simulink model "initial_model1"  (R2017b)
settings: Solver=ode4  StartTime=0.0  StopTime=time_final  FixedStep=time_step  RelTol=1e-3  AbsTol=1e-6
values from neighbouring files (symbols this model uses):
  A_frontal = 2.8    [tesla_sim_data1.m]
  C_d = 0.24    [tesla_sim_data1.m]
  enable_stop = 1    [tesla_sim_data1.m]
  ess_cap_scale = 1    [tesla_sim_data1.m]
  ess_fixtemp = 25    [tesla_sim_data1.m]
  ess_init_soc = soc_init_index(simrun)    [ev_sim_init1.m]
  ess_max_ah_cap = ess_max_kwhr_cap*1000/350*[1 1]    [tesla_sim_data1.m]
  ess_max_volts = 9    [tesla_sim_data1.m]
  ess_min_volts = 6    [tesla_sim_data1.m]
  ess_module_num = 40    [tesla_sim_data1.m]
  ess_r_chg = [ ... (first row only)    [tesla_sim_data1.m]
  ess_r_dis = [ ... (first row only)    [tesla_sim_data1.m]
  ess_res_scale_coef = [1 0 1 0]    [tesla_sim_data1.m]
  ess_res_scale_fun = inline('(x(1)*ess_module_num+x(2))/(x(3)*ess_cap_scale+x(4))','x','ess_module_num','ess_cap_scale')    [tesla_sim_data1.m]
  ess_soc = [0 0.1 0.2 0.3 0.4 0.5 0.6 0.7 0.8 0.9 1]    [tesla_sim_data1.m]
  ess_tmp = [0 25]    [tesla_sim_data1.m]
  ess_voc = [ ... (first row only)    [tesla_sim_data1.m]
  f_rolling = 0.018    [tesla_sim_data1.m]
  FR = 9.73    [tesla_sim_data1.m]
  g_gravity = 9.81    [tesla_sim_data1.m]
  K_factor_in = 2    [ev_sim_init1.m]
  Kp_c = 30    [ev_sim_init1.m]
  m_map_spd = [0	100	250	500	1000	1500	2000	2500	3000	4000	4500	5500	6000	7000	8000	9000	10000]*(2*pi)/60    [tesla_sim_data1.m]
  m_max_trq_IM = min(m_peak_trq_IM, m_peak_pwr*1000./m_map_spd)    [tesla_sim_data1.m]
  m_max_trq_SR = min(m_peak_trq_SR, m_peak_pwr*1000./m_map_spd)    [tesla_sim_data1.m]
  m_min_volts = 200    [tesla_sim_data1.m]
  m_peak_pwr = 310    [tesla_sim_data1.m]
  M_total = (4650+300)/2.2046    (= 2245.3052708)    [tesla_sim_data1.m]
  p00 = -215.8    [tesla_sim_data1.m]
  p01 = 3.368    [tesla_sim_data1.m]
  p02 = -0.0178    [tesla_sim_data1.m]
  p03 = 6.515e-05    [tesla_sim_data1.m]
  p10 = 4.164    [tesla_sim_data1.m]
  p11 = 0.04408    [tesla_sim_data1.m]
  p12 = 9.874e-05    [tesla_sim_data1.m]
  p20 = -0.009417    [tesla_sim_data1.m]
  p21 = 5.981e-06    [tesla_sim_data1.m]
  p30 = 5.161e-06    [tesla_sim_data1.m]
  R_tire = 0.335    [tesla_sim_data1.m]
  regstop_soc = 0.9    [ev_sim_init1.m]
  rho_air = 1.2    [tesla_sim_data1.m]
  Ti_c = 60    [ev_sim_init1.m]
  time_final = 1*length(cyc_mph(:,2))    [ev_sim_init1.m]
  Tt_c = 65    [ev_sim_init1.m]
  v_max_c = 100    [ev_sim_init1.m]
undefined symbols (not defined in the file or in its folder): cyc_mph
libraries: simulink x4
settings Model: ExtModeTrigMode=oneshot  ExtModeArmWhenConnect=off  Creator=sz3lhr  LastModifiedBy=Robert Wygant
settings SolverCC: InitialStep=0.001
settings DataIOCC: SaveFormat=Array  SignalLoggingSaveFormat=ModelDataLogs  SaveOutput=off  SaveTime=off  SignalLoggingName=sigsOut
settings OptimizationCC: BooleanDataType=off  OptimizeBlockIOStorage=off  BufferReuse=off  GlobalBufferReuse=off  ExpressionFolding=off  ExpressionDepthLimit=2147483647  LocalBlockOutputs=off  InitFltsAndDblsToZero=on  LifeSpan=inf
settings DebuggingCC: SaveWithParameterizedLinksMsg=none  UnderspecifiedInitializationDetection=Classic  MergeDetectMultiDrivingBlocksExec=none  SignalResolutionControl=TryResolveAllWithWarning  MultiTaskDSMMsg=warning  MultiTaskCondExecSysMsg=none  FcnCallInpInsideContextMsg=warning  StateNameClashWarn=warning  StrictBusMsg=None  SFUnexpectedBacktrackingDiag=warning  SFNoUnconditionalDefaultTransitionDiag=warning  SFExecutionAtInitializationDiag=none
settings HardwareCC: ProdBitPerPointer=32  ProdBitPerSizeT=32  ProdBitPerPtrDiffT=32  ProdLargestAtomicFloat=None  ProdIntDivRoundTo=Undefined  ProdEndianess=Unspecified  ProdWordSize=32  ProdHWDeviceType=32-bit Generic  TargetUnknown=on
settings ModelReferenceCC: PropagateSignalLabelsOutOfModel=off
settings CodeAppCC: StateflowObjectComments=on
settings GRTTargetCC: TargetFcnLib=ansi_tfl_tmw.mat  TargetLangStandard=C89/C90 (ANSI)  GeneratePreprocessorConditionals=Disable all  CombineOutputUpdateFcns=off  GRTInterface=on
settings ConfigComp: CovMetricSettings=dw  CovHtmlReporting=on  CovSaveCumulativeToWorkspaceVar=on  CovSaveSingleToWorkspaceVar=on  CovExternalEMLEnable=off

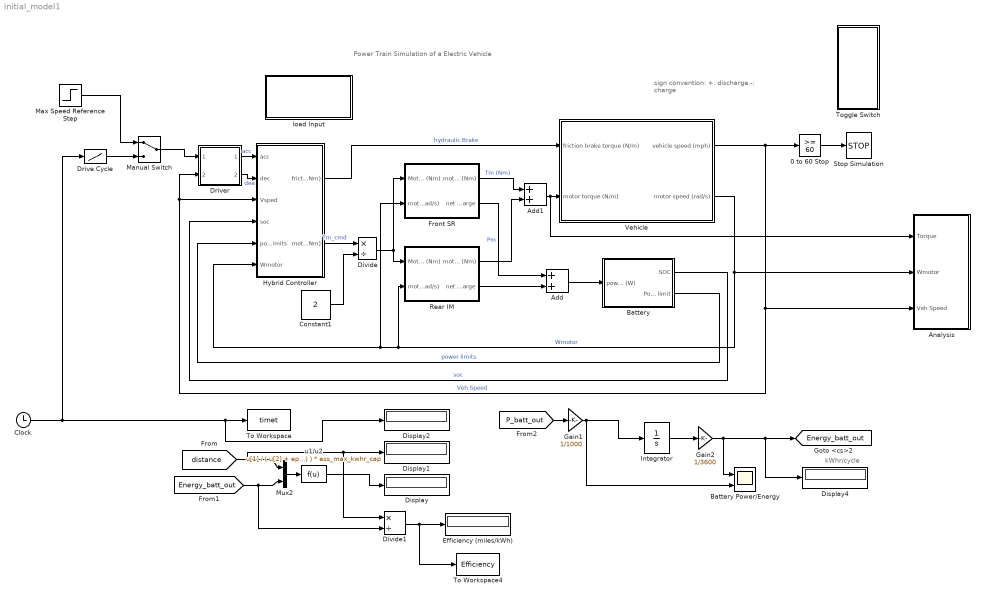
== system initial_model1 ==
  note: Power Train Simulation of a Electric Vehicle
  note: sign convention:
      | +: discharge     -: charge
  note: kWhr/cycle
  0 to 60 Stop : simulink/Logic and Bit Operations/Compare To Constant  relop=>=  const=60  OutDataTypeStr=boolean
  Add : Sum
  Add1 : Sum
  Analysis : Subsystem
  Battery : Subsystem
      mask Display: disp('Battery')
  Battery Power/Energy : Scope  NumInputPorts=2
      settings: Description=Power/Energy
  Clock : Clock
  Constant1 : Constant  Value=2  VectorParams1D=off  SampleTime=-1
  Display{,1..2,4} (4 alike) : Display
  Divide : Product  Inputs=*/
  Divide1 : Product  Inputs=*/
  Drive Cycle : Lookup  InputValues=cyc_mph(:,1)  Table=cyc_mph(:,2)  SaturateOnIntegerOverflow=on
  "Driver " : Subsystem
      mask Display: disp('Driver')
  Efficiency (miles/kWh) : Display
  Front SR : Subsystem
      mask Display: disp('Electric\nMotor')
  Gain1 : Gain  Gain=1/1000  SaturateOnIntegerOverflow=on  OutDataTypeStr=Inherit: Same as input  ParamDataTypeStr=Inherit: Same as input
  Gain2 : Gain  Gain=1/3600  SaturateOnIntegerOverflow=on  OutDataTypeStr=Inherit: Same as input  ParamDataTypeStr=Inherit: Same as input
  Hybrid Controller : Subsystem
      mask Display: disp('Vehicle\nController')
  Integrator : Integrator  LowerSaturationLimit=0
  Manual Switch : ManualSwitch
  Max Speed Reference Step : Step  Time=0.01  After=500  SampleTime=0
  Mux2 : Mux  Inputs=2
  Rear IM : Subsystem
      mask Display: disp('Electric\nMotor')
  Stop Simulation : Stop
  To Workspace : ToWorkspace  VariableName=timet  SampleTime=-1
  To Workspace4 : ToWorkspace  VariableName=Efficiency  SampleTime=-1
      settings: Save2DSignal=2-D array (concatenate along first dimension)
  Toggle Switch : Subsystem  DialogController=hmiCreateDDGDialog  IsWebBlock=on  mask(MWDashboardBlock){webBlockId=bcc0d4d4-d3e6-44b1-9da5-97979c717e77, webBlockType=toggleswitch, ShowInLibBrowser=on, ShowInitialText=on, HMISrcModelName=initial_model1}
      mask prompts: webBlockId "WebBlock Id"; webBlockType "WebBlock Type"; HMISrcModelName "Source Model"
      mask help: SimulinkHMI:dialogs:SwitchDialogDesc
      mask Help: helpview([docroot '/mapfiles/simulink.map'], 'hmi_toggle_switch')
      mask Display:
      | if strcmp(get_param(bdroot(gcb),'BlockDiagramType'), 'library')
      |     image([(matlabroot) '/toolbox/simulink/hmi/icons/ToggleSwitch.png']);
      | end
  Vehicle : Subsystem
      mask Display: disp('Vehicle \nDynamic Model')
  load Input : Subsystem
      settings: OpenFcn=ev_sim_init
      mask Help: This block runs/ndes_init.m file in the main directory
      mask Display: disp('Load Input Data\nRun Simulation')
  u1/u2 : Fcn  Expr=u[1] / ( u[2] + eps*(u[2] == 0) ) * ess_max_kwhr_cap
  tag scope: Energy_batt_out=global
  wires:
  Battery/1(SOC) -> Hybrid Controller/4(soc)  "soc"
  Hybrid Controller/1(friction brake torque (Nm)) -> Vehicle/1(friction brake torque (N/m))  "hydraulic Brake"
  Vehicle/1(vehicle speed (mph)) -> 0 to 60 Stop/1, Analysis/3(Veh Speed), Hybrid Controller/3(Vsped), "Driver "/2(Velocity (mph))  "Veh Speed"
  "Driver "/1(Accel Comd) -> Hybrid Controller/1(acc)  "acc"
  "Driver "/2(Brake Comd) -> Hybrid Controller/2(dec)  "dea"
  Vehicle/2(motor speed (rad/s)) -> Analysis/2(Wmotor), Rear IM/2(motor speed (rad/s)), Front SR/2(motor speed (rad/s)), Hybrid Controller/6(Wmotor)  "Wmotor"
  Battery/2(Power limit) -> Hybrid Controller/5(power limits)  "power limits"
  Clock/1 -> Drive Cycle/1, To Workspace/1, Display2/1
  [distance] -> Divide1/1, Display1/1, Mux2/1
  [Energy_batt_out] -> Divide1/2, Mux2/2
  u1/u2/1 -> Display/1
  Mux2/1 -> u1/u2/1
  [P_batt_out] -> Gain1/1
  Gain1/1 -> Integrator/1, Battery Power/Energy/2
  Integrator/1 -> Gain2/1
  Gain2/1 -> [Energy_batt_out], Display4/1, Battery Power/Energy/1
  0 to 60 Stop/1 -> Stop Simulation/1
  Add/1 -> Battery/1(power req'd into bus (W))
  Rear IM/2(net Power >0 discharge <0 charge) -> Add/2
  Front SR/2(net Power >0 discharge <0 charge) -> Add/1  "Pm"
  Rear IM/1(motor torque output (Nm)) -> Add1/2
  Front SR/1(motor torque output (Nm)) -> Add1/1  "Tm (Nm)"
  Hybrid Controller/2(motor torque command (Nm)) -> Divide/1  "Tm_cmd"
  Constant1/1 -> Divide/2
  Divide/1 -> Rear IM/1(Motor demand Torque (Nm)), Front SR/1(Motor demand Torque (Nm))
  Add1/1 -> Analysis/1(Torque), Vehicle/2(motor torque (N/m))
  Max Speed Reference Step/1 -> Manual Switch/1
  Drive Cycle/1 -> Manual Switch/2
  Manual Switch/1 -> "Driver "/1(speed_desired)
  Divide1/1 -> To Workspace4/1, Efficiency (miles/kWh)/1

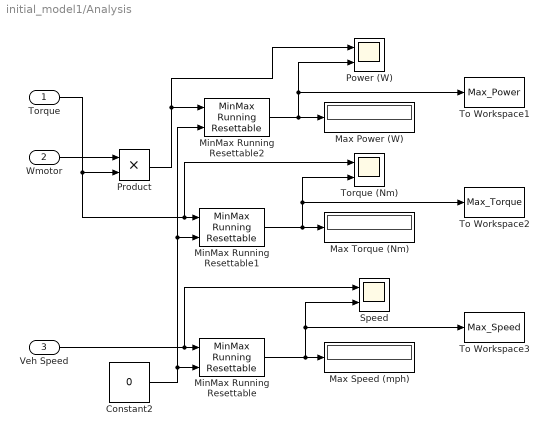
== system initial_model1/Analysis ==
  Torque : Inport
  Wmotor : Inport  Port=2
  Veh Speed : Inport  Port=3
  Constant2 : Constant  Value=0  VectorParams1D=off  SampleTime=-1
  Max Power (W) : Display
  Max Speed (mph) : Display
  Max Torque (Nm) : Display
  MinMax Running Resettable : simulink/Math Operations/MinMax Running Resettable  Function=max  vinit=0.0
  MinMax Running Resettable1 : simulink/Math Operations/MinMax Running Resettable  Function=max  vinit=0.0
  MinMax Running Resettable2 : simulink/Math Operations/MinMax Running Resettable  Function=max  vinit=0.0
  Power (W) : Scope  NumInputPorts=2
  Product : Product
  Speed : Scope  NumInputPorts=2
  To Workspace1 : ToWorkspace  VariableName=Max_Power  SampleTime=-1
      settings: Save2DSignal=2-D array (concatenate along first dimension)
  To Workspace2 : ToWorkspace  VariableName=Max_Torque  SampleTime=-1
      settings: Save2DSignal=2-D array (concatenate along first dimension)
  To Workspace3 : ToWorkspace  VariableName=Max_Speed  SampleTime=-1
      settings: Save2DSignal=2-D array (concatenate along first dimension)
  Torque (Nm) : Scope  NumInputPorts=2
  wires:
  Veh Speed/1 -> Speed/1, MinMax Running Resettable/1
  Wmotor/1 -> Product/1
  Torque/1 -> Torque (Nm)/1, MinMax Running Resettable1/1, Product/2
  Product/1 -> MinMax Running Resettable2/1, Power (W)/1
  Constant2/1 -> MinMax Running Resettable2/2, MinMax Running Resettable1/2, MinMax Running Resettable/2
  MinMax Running Resettable1/1 -> To Workspace2/1, Torque (Nm)/2, Max Torque (Nm)/1
  MinMax Running Resettable/1 -> To Workspace3/1, Speed/2, Max Speed (mph)/1
  MinMax Running Resettable2/1 -> To Workspace1/1, Power (W)/2, Max Power (W)/1

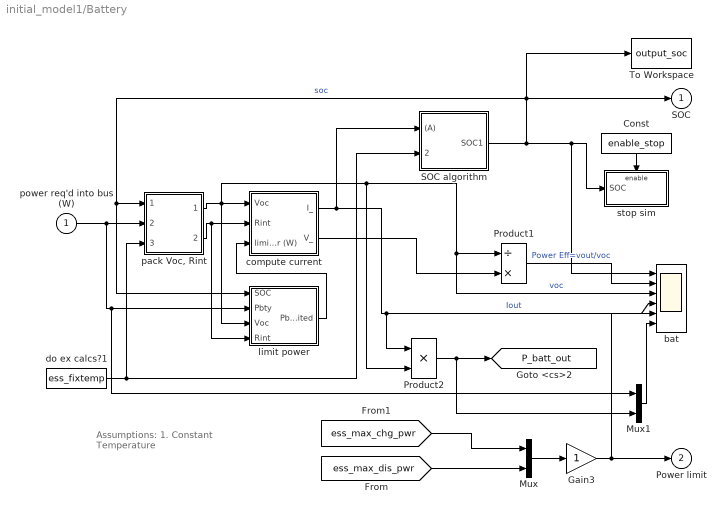
== system initial_model1/Battery ==
  note: Assumptions:
      | 1. Constant Temperature
  power req'd into bus (W) : Inport
  Const : Constant  Value=enable_stop
  Gain3 : Gain  SaturateOnIntegerOverflow=on  OutDataTypeStr=Inherit: Same as input  ParamDataTypeStr=Inherit: Same as input
  Mux : Mux  Inputs=2
  Mux1 : Mux  Inputs=2
  Product1 : Product  Inputs=/*  SaturateOnIntegerOverflow=on  InputSameDT=on  OutDataTypeStr=Inherit: Same as first input
  Product2 : Product  Inputs=**  SaturateOnIntegerOverflow=on  InputSameDT=on  OutDataTypeStr=Inherit: Same as first input
  SOC algorithm : Subsystem  AncestorBlock=|
      | lib_energy_storage/Ess Choices/energy
      | storage <ess>/SOC
      | algorithm
      mask Display: disp('SOC\nalgorithm')
  To Workspace : ToWorkspace  VariableName=output_soc  SampleTime=-1
  bat : Scope  NumInputPorts=6
  compute current : Subsystem  AncestorBlock=|
      | lib_energy_storage/Ess Choices/energy
      | storage <ess>/compute
      | current
      mask Display: disp('Compute\nCurrent')
  do ex calcs?1 : Constant  Value=ess_fixtemp
  limit power : Subsystem  AncestorBlock=lib_energy_storage/Ess Choices/energy storage <ess>/limit power
      mask Display: disp('Limit\nPower')
  "pack Voc, Rint" : Subsystem  AncestorBlock=|
      | lib_energy_storage/Ess Choices/energy
      | storage <ess>/pack
      | Voc, Rint
      mask Display: disp('Pack\nVoc,Rint')
  stop sim : Subsystem  AncestorBlock=lib_energy_storage/Ess Choices/energy storage <ess>/stop sim  TreatAsAtomicUnit=on
  SOC : Outport  InitialOutput=0
  Power limit : Outport  Port=2  InitialOutput=0
  tag scope: P_batt_out=global
  wires:
  limit power/1("Pbty, limited") -> compute current/3(limited output power (W))
  "pack Voc, Rint"/1(pack open- circuit voltage) -> limit power/3(Voc), compute current/1(Voc), Product1/1, bat/3, Product2/2  "voc"
  "pack Voc, Rint"/2(pack resistance) -> compute current/2(Rint), limit power/4(Rint)
  Const/1 -> stop sim/Enable
  SOC algorithm/1(SOC1) -> limit power/1(SOC), "pack Voc, Rint"/1(SOC (prev)), SOC/1, To Workspace/1, stop sim/1(SOC), bat/1  "soc"
  compute current/1(I_) -> SOC algorithm/1((A)), Product2/1, bat/4  "Iout"
  power req'd into bus (W)/1 -> "pack Voc, Rint"/2(req'd battery power (W)), limit power/2(Pbty), Mux1/1
  compute current/2(V_) -> Product1/2
  do ex calcs?1/1 -> "pack Voc, Rint"/3(mod tmp (C)), SOC algorithm/2(tmp (C))
  Mux/1 -> Gain3/1
  Product1/1 -> bat/2  "Power Eff=vout/voc"
  [ess_max_dis_pwr] -> Mux/2
  [ess_max_chg_pwr] -> Mux/1
  Gain3/1 -> Power limit/1, bat/5
  Product2/1 -> [P_batt_out], Mux1/2
  Mux1/1 -> bat/6

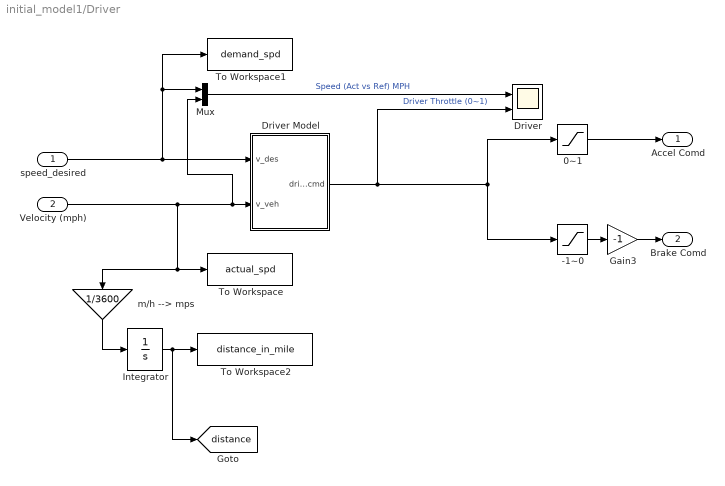
== system initial_model1/Driver  ==
  speed_desired : Inport
  Velocity (mph) : Inport  Port=2
  -1~0 : Saturate  UpperLimit=0  LowerLimit=-1
  0~1 : Saturate  UpperLimit=1  LowerLimit=0
  Driver : Scope  NumInputPorts=2
  Driver Model : Subsystem
  Gain3 : Gain  Gain=-1  SaturateOnIntegerOverflow=on  OutDataTypeStr=Inherit: Same as input  ParamDataTypeStr=Inherit: Same as input
  Integrator : Integrator  LowerSaturationLimit=0
  Mux : Mux  Inputs=2
  To Workspace : ToWorkspace  VariableName=actual_spd  SampleTime=-1
  To Workspace1 : ToWorkspace  VariableName=demand_spd  SampleTime=-1
  To Workspace2 : ToWorkspace  VariableName=distance_in_mile  SampleTime=time_final
  m/h --> mps : Gain  Gain=1/3600  SaturateOnIntegerOverflow=on  OutDataTypeStr=Inherit: Same as input  ParamDataTypeStr=Inherit: Same as input
  Accel Comd : Outport  InitialOutput=0
  Brake Comd : Outport  Port=2  InitialOutput=0
  tag scope: distance=global
  wires:
  speed_desired/1 -> Driver Model/1(v_des), To Workspace1/1, Mux/1
  Velocity (mph)/1 -> To Workspace/1, m/h --> mps/1, Driver Model/2(v_veh), Mux/2
  Driver Model/1(driver_cmd) -> Driver/2, 0~1/1, -1~0/1  "Driver Throttle (0~1)"
  -1~0/1 -> Gain3/1
  0~1/1 -> Accel Comd/1
  Gain3/1 -> Brake Comd/1
  Mux/1 -> Driver/1  "Speed (Act vs Ref) MPH"
  Integrator/1 -> To Workspace2/1, [distance]
  m/h --> mps/1 -> Integrator/1

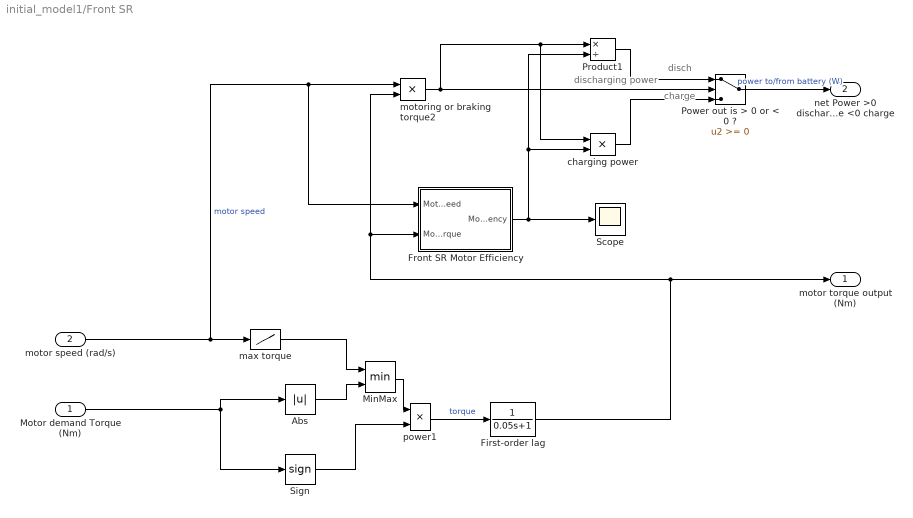
== system initial_model1/Front SR ==
  note: disch
  note: charge
  note: discharging
      | power
  Motor demand Torque (Nm) : Inport
  motor speed (rad/s) : Inport  Port=2
  Abs : Abs  SaturateOnIntegerOverflow=on
  First-order lag : TransferFcn  Denominator=[0.05 1]
  Front SR Motor Efficiency : Subsystem
      mask Display:
      | color('green')
      | disp("Motor Efficiency")
  MinMax : MinMax  Inputs=2  SaturateOnIntegerOverflow=on  InputSameDT=on
  Power out is > 0 or < 0 ? : Switch  SaturateOnIntegerOverflow=on  InputSameDT=on
  Product1 : Product  Inputs=*/  SaturateOnIntegerOverflow=on  InputSameDT=on  OutDataTypeStr=Inherit: Same as first input
  Scope : Scope
  Sign : Signum
  charging power : Product  SaturateOnIntegerOverflow=on  InputSameDT=on  OutDataTypeStr=Inherit: Same as first input
  max torque : Lookup  InputValues=m_map_spd  Table=m_max_trq_SR  SaturateOnIntegerOverflow=on
  motoring or braking torque2 : Product  SaturateOnIntegerOverflow=on  InputSameDT=on  OutDataTypeStr=Inherit: Same as first input
  power1 : Product  SaturateOnIntegerOverflow=on  InputSameDT=on  OutDataTypeStr=Inherit: Same as first input
  motor torque output (Nm) : Outport  InitialOutput=0
  net Power >0 discharge <0 charge : Outport  Port=2  InitialOutput=0
  wires:
  charging power/1 -> Power out is > 0 or < 0 ?/3
  Product1/1 -> Power out is > 0 or < 0 ?/1
  Power out is > 0 or < 0 ?/1 -> net Power >0 discharge <0 charge/1  "power to/from battery (W)"
  Motor demand Torque (Nm)/1 -> Sign/1, Abs/1
  power1/1 -> First-order lag/1  "torque"
  motoring or braking torque2/1 -> Product1/1, charging power/1, Power out is > 0 or < 0 ?/2
  Abs/1 -> MinMax/2
  MinMax/1 -> power1/1
  Sign/1 -> power1/2
  motor speed (rad/s)/1 -> max torque/1, Front SR Motor Efficiency/1(Motor_speed), motoring or braking torque2/1  "motor speed"
  First-order lag/1 -> motor torque output (Nm)/1, Front SR Motor Efficiency/2(Motor_torque), motoring or braking torque2/2
  max torque/1 -> MinMax/1
  Front SR Motor Efficiency/1(Motor_efficiency) -> Scope/1, charging power/2, Product1/2

== system initial_model1/Hybrid Controller ==
  acc : Inport
  dec : Inport  Port=2
  Vsped : Inport  Port=3
  soc : Inport  Port=4
  power limits : Inport  Port=5
  Wmotor : Inport  Port=6
  Brake : Subsystem  AncestorBlock=|
      | lib_controls/<vc> prius/Coordinated
      |  Controller/max engine
      | efficiency point
      mask Display: disp('Braking\nControl')
  Demux : Demux  Outputs=2
  Drive : Subsystem  AncestorBlock=|
      | lib_controls/<vc> prius/Coordinated
      |  Controller/max engine
      | efficiency point
      mask Display: disp('Driving\nControl')
  Mux : Mux  Inputs=2
  Mux1 : Mux  Inputs=2
  power >=0 drive <0 brake : Switch  SaturateOnIntegerOverflow=on
  pwr_demand : Subsystem
      mask Display: disp('Power\nDemand')
  friction brake torque (Nm) : Outport
  motor torque command (Nm) : Outport  Port=2
  wires:
  pwr_demand/1(pwr dmd (W)) -> Drive/1(pwr requested), Brake/1(Driver power requested (W)), power >=0 drive <0 brake/2
  acc/1 -> pwr_demand/1(Accel cmd)
  dec/1 -> pwr_demand/2(Decel cmd)
  Mux/1 -> power >=0 drive <0 brake/1
  Mux1/1 -> power >=0 drive <0 brake/3
  power >=0 drive <0 brake/1 -> Demux/1
  Vsped/1 -> Brake/2(Veh speed (mph))
  soc/1 -> Brake/3(soc)
  power limits/1 -> Brake/4(Power limit (W)), Drive/2(Power limits (W))
  Wmotor/1 -> Brake/5(motor speed(rad/s)), Drive/3(motor speed (rad/s))
  Drive/2(motor torque command (Nm)) -> Mux/2
  Drive/1(friction brake torque (Nm)) -> Mux/1
  Brake/1(friction brake torque command (Nm)) -> Mux1/1
  Brake/2(motor torque command (Nm)) -> Mux1/2
  Demux/2 -> motor torque command (Nm)/1
  Demux/1 -> friction brake torque (Nm)/1

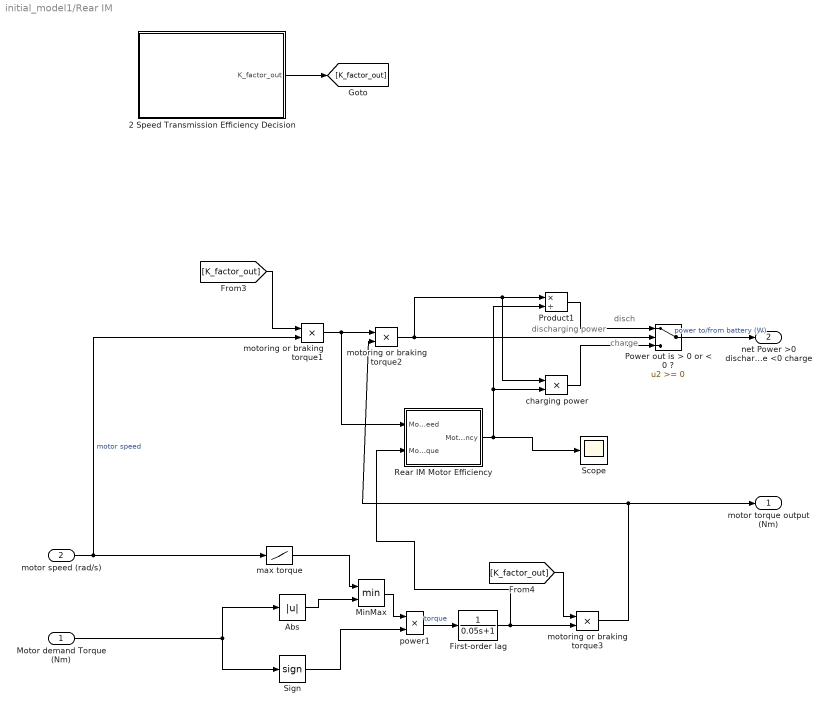
== system initial_model1/Rear IM ==
  note: disch
  note: charge
  note: discharging
      | power
  Motor demand Torque (Nm) : Inport
  motor speed (rad/s) : Inport  Port=2
  2 Speed Transmission Efficiency Decision : Subsystem
  Abs : Abs  SaturateOnIntegerOverflow=on
  First-order lag : TransferFcn  Denominator=[0.05 1]
  MinMax : MinMax  Inputs=2  SaturateOnIntegerOverflow=on  InputSameDT=on
  Power out is > 0 or < 0 ? : Switch  SaturateOnIntegerOverflow=on  InputSameDT=on
  Product1 : Product  Inputs=*/  SaturateOnIntegerOverflow=on  InputSameDT=on  OutDataTypeStr=Inherit: Same as first input
  Rear IM Motor Efficiency : Subsystem
      mask Display:
      | color('green')
      | disp("Motor Efficiency")
  Scope : Scope
  Sign : Signum
  charging power : Product  SaturateOnIntegerOverflow=on  InputSameDT=on  OutDataTypeStr=Inherit: Same as first input
  max torque : Lookup  InputValues=m_map_spd  Table=m_max_trq_IM  SaturateOnIntegerOverflow=on
  motoring or braking torque1 : Product  SaturateOnIntegerOverflow=on  InputSameDT=on  OutDataTypeStr=Inherit: Same as first input
  motoring or braking torque2 : Product  SaturateOnIntegerOverflow=on  InputSameDT=on  OutDataTypeStr=Inherit: Same as first input
  motoring or braking torque3 : Product  SaturateOnIntegerOverflow=on  InputSameDT=on  OutDataTypeStr=Inherit: Same as first input
  power1 : Product  SaturateOnIntegerOverflow=on  InputSameDT=on  OutDataTypeStr=Inherit: Same as first input
  motor torque output (Nm) : Outport  InitialOutput=0
  net Power >0 discharge <0 charge : Outport  Port=2  InitialOutput=0
  wires:
  charging power/1 -> Power out is > 0 or < 0 ?/3
  Product1/1 -> Power out is > 0 or < 0 ?/1
  Power out is > 0 or < 0 ?/1 -> net Power >0 discharge <0 charge/1  "power to/from battery (W)"
  motor speed (rad/s)/1 -> max torque/1, motoring or braking torque1/2  "motor speed"
  Motor demand Torque (Nm)/1 -> Abs/1, Sign/1
  power1/1 -> First-order lag/1  "torque"
  motoring or braking torque2/1 -> Product1/1, charging power/1, Power out is > 0 or < 0 ?/2
  Abs/1 -> MinMax/2
  MinMax/1 -> power1/1
  Sign/1 -> power1/2
  max torque/1 -> MinMax/1
  First-order lag/1 -> Rear IM Motor Efficiency/2(Motor_torque), motoring or braking torque3/2
  motoring or braking torque1/1 -> Rear IM Motor Efficiency/1(Motor_speed), motoring or braking torque2/1
  motoring or braking torque3/1 -> motoring or braking torque2/2, motor torque output (Nm)/1
  2 Speed Transmission Efficiency Decision/1(K_factor_out) -> [K_factor_out]
  [K_factor_out] -> motoring or braking torque1/1
  [K_factor_out] -> motoring or braking torque3/1
  Rear IM Motor Efficiency/1(Motor_efficiency) -> charging power/2, Product1/2, Scope/1

== system initial_model1/Toggle Switch ==

== system initial_model1/Vehicle ==
  friction brake torque (N/m) : Inport
  motor torque (N/m) : Inport  Port=2
  Dynamics : Subsystem
      mask Display: disp('Vehicle \nDynamic Model')
  rad/s --> mph : Gain  Gain=R_tire/1000*0.621371*3600  SaturateOnIntegerOverflow=on  OutDataTypeStr=Inherit: Same as input  ParamDataTypeStr=Inherit: Same as input
  w_r->w_wh : Fcn  Expr=u/FR
  vehicle speed (mph) : Outport
  motor speed (rad/s) : Outport  Port=2
  wires:
  motor torque (N/m)/1 -> Dynamics/2(Tm: motor torque (N/m))
  friction brake torque (N/m)/1 -> Dynamics/3("Tfb: friction brake torque (N/m) ")
  w_r->w_wh/1 -> Dynamics/1(wheel speed (rad/s)), rad/s --> mph/1
  rad/s --> mph/1 -> vehicle speed (mph)/1
  Dynamics/1(motor speed (rad/s)) -> motor speed (rad/s)/1, w_r->w_wh/1

== system initial_model1/load Input ==
  note: double_click to load

== system initial_model1/Battery/SOC algorithm ==
  note: SOC=(Max Ah capacity-Ah used)/Max Ah capacity
  (A) : Inport
  tmp (C) : Inport  Port=2
  (sec->hrs) : Gain  Gain=1/3600  SaturateOnIntegerOverflow=on  OutDataTypeStr=Inherit: Same as input  ParamDataTypeStr=Inherit: Same as input
  0 <= SOC <= 1 : Saturate  UpperLimit=1  LowerLimit=0
  A-h remaining : Sum  Inputs=-+  SaturateOnIntegerOverflow=on  InputSameDT=on  OutDataTypeStr=Inherit: Same as first input
  Ah used : Integrator  InitialConditionSource=external  InitialCondition=(1-ess_init_soc)*ess_max_ah_cap
  Fcn : Fcn  Expr=1/u
  Fcn1 : Fcn  Expr=(1-ess_init_soc)*u
  SOC : Product  SaturateOnIntegerOverflow=on  InputSameDT=on  OutDataTypeStr=Inherit: Same as first input
  max cap : Lookup  InputValues=ess_tmp  Table=ess_max_ah_cap*ess_cap_scale  SaturateOnIntegerOverflow=on
  SOC1 : Outport  InitialOutput=0
  wires:
  (A)/1 -> (sec->hrs)/1
  (sec->hrs)/1 -> Ah used/1
  Ah used/1 -> A-h remaining/1
  Fcn/1 -> SOC/2
  SOC/1 -> 0 <= SOC <= 1/1
  A-h remaining/1 -> SOC/1
  0 <= SOC <= 1/1 -> SOC1/1
  tmp (C)/1 -> max cap/1
  max cap/1 -> A-h remaining/2, Fcn/1, Fcn1/1
  Fcn1/1 -> Ah used/2

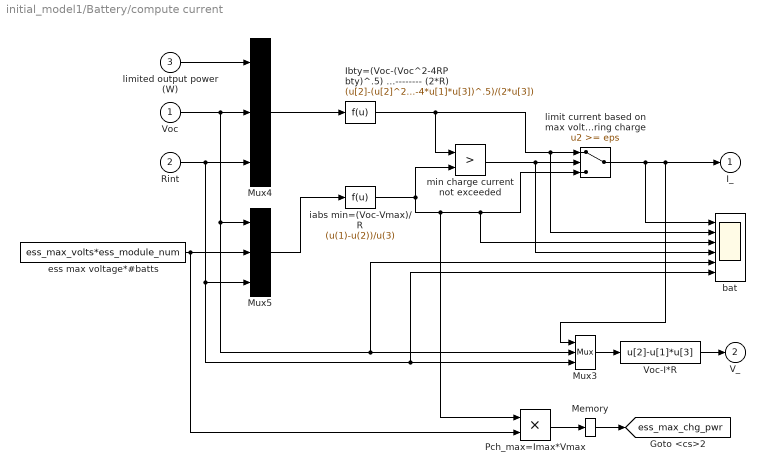
== system initial_model1/Battery/compute current ==
  Voc : Inport
  Rint : Inport  Port=2
  limited output power (W) : Inport  Port=3
  Ibty=(Voc-(Voc^2-4RPbty)^.5) ----------------------------- (2*R) : Fcn  Expr=(u[2]-(u[2]^2-4*u[1]*u[3])^.5)/(2*u[3])
  Memory : Memory
  Mux3 : Mux  Inputs=3
  Mux4 : Mux  Inputs=3
  Mux5 : Mux  Inputs=3
  Pch_max=Imax*Vmax : Product  SaturateOnIntegerOverflow=on  InputSameDT=on  OutDataTypeStr=Inherit: Same as first input
  Voc-I*R : Fcn  Expr=u[2]-u[1]*u[3]
  bat : Scope  NumInputPorts=6
  ess max voltage*#batts : Constant  Value=ess_max_volts*ess_module_num
  iabs min=(Voc-Vmax)/R : Fcn  Expr=(u(1)-u(2))/u(3)
  limit current based on max voltage during charge : Switch  Threshold=eps  SaturateOnIntegerOverflow=on  InputSameDT=on
  min charge current not exceeded : RelationalOperator  Operator=>  RndMeth=Nearest  InputSameDT=on
  I_ : Outport  InitialOutput=0
  V_ : Outport  Port=2  InitialOutput=0
  tag scope: ess_max_chg_pwr=global
  wires:
  limited output power (W)/1 -> Mux4/1
  Voc/1 -> Mux4/2, Mux5/1, Mux3/2, bat/5
  Rint/1 -> Mux4/3, Mux5/3, Mux3/3, bat/6
  Ibty=(Voc-(Voc^2-4RPbty)^.5) ----------------------------- (2*R)/1 -> min charge current not exceeded/1, limit current based on max voltage during charge/1, bat/2
  iabs min=(Voc-Vmax)/R/1 -> min charge current not exceeded/2, Pch_max=Imax*Vmax/1, limit current based on max voltage during charge/3, bat/3
  limit current based on max voltage during charge/1 -> Mux3/1, I_/1, bat/1
  min charge current not exceeded/1 -> limit current based on max voltage during charge/2, bat/4
  Mux3/1 -> Voc-I*R/1
  Voc-I*R/1 -> V_/1
  Mux4/1 -> Ibty=(Voc-(Voc^2-4RPbty)^.5) ----------------------------- (2*R)/1
  Mux5/1 -> iabs min=(Voc-Vmax)/R/1
  ess max voltage*#batts/1 -> Mux5/2, Pch_max=Imax*Vmax/2
  Pch_max=Imax*Vmax/1 -> Memory/1
  Memory/1 -> [ess_max_chg_pwr]

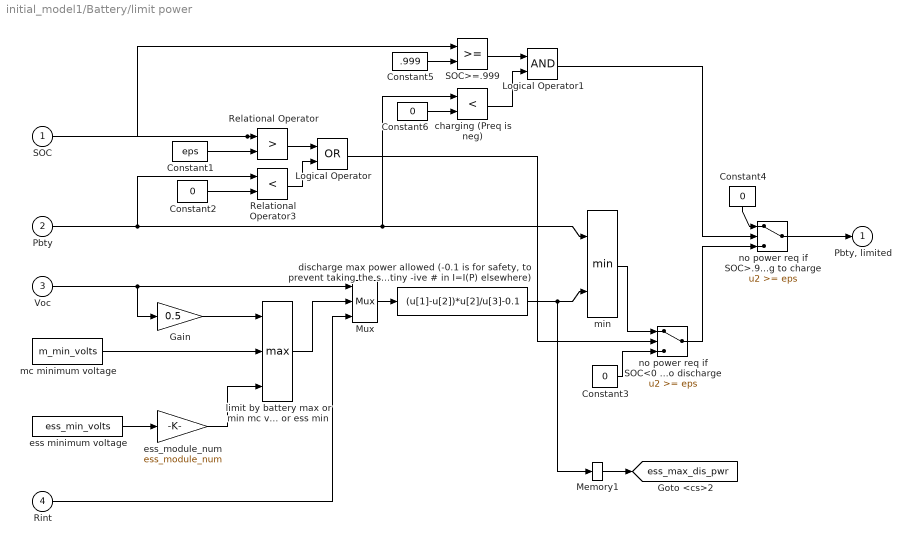
== system initial_model1/Battery/limit power ==
  SOC : Inport
  Pbty : Inport  Port=2
  Voc : Inport  Port=3
  Rint : Inport  Port=4
  Constant1 : Constant  Value=eps
  Constant{2..4,6} (4 alike) : Constant  Value=0
  Constant5 : Constant  Value=.999
  Gain : Gain  Gain=0.5  SaturateOnIntegerOverflow=on  OutDataTypeStr=Inherit: Same as input  ParamDataTypeStr=Inherit: Same as input
  Logical Operator : Logic  Operator=OR
  Logical Operator1 : Logic
  Memory1 : Memory
  Mux : Mux  Inputs=3
  Relational Operator : RelationalOperator  Operator=>  RndMeth=Nearest  InputSameDT=on
  Relational Operator3 : RelationalOperator  Operator=<  RndMeth=Nearest  InputSameDT=on
  SOC>=.999 : RelationalOperator  RndMeth=Nearest  InputSameDT=on
  charging (Preq is neg) : RelationalOperator  Operator=<  RndMeth=Nearest  InputSameDT=on
  "discharge max power allowed (-0.1 is for safety, to prevent taking the square of a tiny -ive # in I=I(P) elsewhere)" : Fcn  Expr=(u[1]-u[2])*u[2]/u[3]-0.1
  ess minimum voltage : Constant  Value=ess_min_volts
  ess_module_num : Gain  Gain=ess_module_num  SaturateOnIntegerOverflow=on  OutDataTypeStr=Inherit: Same as input  ParamDataTypeStr=Inherit: Same as input
  limit by battery max or min mc voltage or ess min : MinMax  Function=max  Inputs=3  SaturateOnIntegerOverflow=on  InputSameDT=on
  mc minimum voltage : Constant  Value=m_min_volts
  min : MinMax  Inputs=2  SaturateOnIntegerOverflow=on  InputSameDT=on
  no power req if SOC<0 and trying to discharge : Switch  Threshold=eps  SaturateOnIntegerOverflow=on  InputSameDT=on
  no power req if SOC>.999 and trying to charge : Switch  Threshold=eps  SaturateOnIntegerOverflow=on  InputSameDT=on
  "Pbty, limited" : Outport  InitialOutput=0
  tag scope: ess_max_dis_pwr=global
  wires:
  Constant1/1 -> Relational Operator/2
  Relational Operator/1 -> Logical Operator/1
  Pbty/1 -> Relational Operator3/1, charging (Preq is neg)/1, min/1
  Constant2/1 -> Relational Operator3/2
  Relational Operator3/1 -> Logical Operator/2
  Constant3/1 -> no power req if SOC<0 and trying to discharge/3
  Logical Operator/1 -> no power req if SOC<0 and trying to discharge/2
  Voc/1 -> Mux/1, Gain/1
  min/1 -> no power req if SOC<0 and trying to discharge/1
  Mux/1 -> "discharge max power allowed (-0.1 is for safety, to prevent taking the square of a tiny -ive # in I=I(P) elsewhere)"/1
  limit by battery max or min mc voltage or ess min/1 -> Mux/2
  "discharge max power allowed (-0.1 is for safety, to prevent taking the square of a tiny -ive # in I=I(P) elsewhere)"/1 -> min/2, Memory1/1
  mc minimum voltage/1 -> limit by battery max or min mc voltage or ess min/2
  Rint/1 -> Mux/3
  Gain/1 -> limit by battery max or min mc voltage or ess min/1
  ess minimum voltage/1 -> ess_module_num/1
  ess_module_num/1 -> limit by battery max or min mc voltage or ess min/3
  SOC/1 -> Relational Operator/1, SOC>=.999/1
  SOC>=.999/1 -> Logical Operator1/1
  Constant6/1 -> charging (Preq is neg)/2
  charging (Preq is neg)/1 -> Logical Operator1/2
  Constant5/1 -> SOC>=.999/2
  Constant4/1 -> no power req if SOC>.999 and trying to charge/1
  no power req if SOC<0 and trying to discharge/1 -> no power req if SOC>.999 and trying to charge/3
  no power req if SOC>.999 and trying to charge/1 -> "Pbty, limited"/1
  Logical Operator1/1 -> no power req if SOC>.999 and trying to charge/2
  Memory1/1 -> [ess_max_dis_pwr]

== system initial_model1/Battery/pack Voc, Rint ==
  SOC (prev) : Inport
  req'd battery power (W) : Inport  Port=2
  mod tmp (C) : Inport  Port=3
  #bty : Constant  Value=ess_module_num
  Product : Product  SaturateOnIntegerOverflow=on  InputSameDT=on  OutDataTypeStr=Inherit: Same as first input
  Rchg (ohms) : Subsystem  mask(2-D Table Lookup){xindex=ess_tmp, yindex=ess_soc, table=ess_r_chg}
      mask prompts: xindex "X Index"; yindex "Y Index"
      mask help:
      | Two Dimensional Table Lookup
      | The first input corresponds to X Index and the second input corresponds to the Y Index
      mask init:
      | sftab2chk(xindex,yindex,table);
      mask Help: This block returns a linearly interpolated intersection from the table using the X index (which corresponds to the rows of the table) and the Y index (which corresponds to the columns of the table).  Extrapolation is used.
      mask Display: plot(-10,-10,110,110,[90,50,10],[90,40,30],[90,50,10],[50,26,20],[90,50,10],[22,13,10])
  Rdis (ohms) : Subsystem  mask(2-D Table Lookup){xindex=ess_tmp, yindex=ess_soc, table=ess_r_dis}
      mask prompts: xindex "X Index"; yindex "Y Index"
      mask help:
      | Two Dimensional Table Lookup
      | The first input corresponds to X Index and the second input corresponds to the Y Index
      mask init:
      | sftab2chk(xindex,yindex,table);
      mask Help: This block returns a linearly interpolated intersection from the table using the X index (which corresponds to the rows of the table) and the Y index (which corresponds to the columns of the table).  Extrapolation is used.
      mask Display: plot(-10,-10,110,110,[90,50,10],[90,40,30],[90,50,10],[50,26,20],[90,50,10],[22,13,10])
  Switch : Switch  SaturateOnIntegerOverflow=on  InputSameDT=on
  VOC (V) : Subsystem  mask(2-D Table Lookup){xindex=ess_tmp, yindex=ess_soc, table=ess_voc}
      mask prompts: xindex "X Index"; yindex "Y Index"
      mask help:
      | Two Dimensional Table Lookup
      | The first input corresponds to X Index and the second input corresponds to the Y Index
      mask init:
      | sftab2chk(xindex,yindex,table);
      mask Help: This block returns a linearly interpolated intersection from the table using the X index (which corresponds to the rows of the table) and the Y index (which corresponds to the columns of the table).  Extrapolation is used.
      mask Display: plot(-10,-10,110,110,[90,50,10],[90,40,30],[90,50,10],[50,26,20],[90,50,10],[22,13,10])
  resistance scale fun : Gain  Gain=ess_res_scale_fun(ess_res_scale_coef,ess_module_num,ess_cap_scale)  SaturateOnIntegerOverflow=on  OutDataTypeStr=Inherit: Same as input  ParamDataTypeStr=Inherit: Same as input
  resistance scale fun1 : Gain  Gain=ess_res_scale_fun(ess_res_scale_coef,ess_module_num,ess_cap_scale)  SaturateOnIntegerOverflow=on  OutDataTypeStr=Inherit: Same as input  ParamDataTypeStr=Inherit: Same as input
  pack open- circuit voltage : Outport  InitialOutput=0
  pack resistance : Outport  Port=2  InitialOutput=0
  wires:
  Rchg (ohms)/1(table out) -> resistance scale fun1/1
  Rdis (ohms)/1(table out) -> resistance scale fun/1
  Switch/1 -> pack resistance/1
  #bty/1 -> Product/2
  Product/1 -> pack open- circuit voltage/1
  VOC (V)/1(table out) -> Product/1
  req'd battery power (W)/1 -> Switch/2
  SOC (prev)/1 -> VOC (V)/2(y0), Rdis (ohms)/2(y0), Rchg (ohms)/2(y0)
  mod tmp (C)/1 -> VOC (V)/1(x0), Rdis (ohms)/1(x0), Rchg (ohms)/1(x0)
  resistance scale fun1/1 -> Switch/3
  resistance scale fun/1 -> Switch/1

== system initial_model1/Battery/stop sim ==
  SOC : Inport
  Enable : EnablePort
  Const : Constant  Value=.001
  Relational Operator : RelationalOperator  Operator=<  RndMeth=Nearest  InputSameDT=on
  Stop Simulation : Stop
  wires:
  Const/1 -> Relational Operator/2
  SOC/1 -> Relational Operator/1
  Relational Operator/1 -> Stop Simulation/1

== system initial_model1/Driver /Driver Model ==
  v_des : Inport
  v_veh : Inport  Port=2
  "-1 to 1 " : Saturate  UpperLimit=1  LowerLimit=-1
  1/Ti_c : Gain  Gain=1/Ti_c  SaturateOnIntegerOverflow=on  OutDataTypeStr=Inherit: Same as input  ParamDataTypeStr=Inherit: Same as input
  1/Tt_c : Gain  Gain=1/Tt_c  SaturateOnIntegerOverflow=on  OutDataTypeStr=Inherit: Same as input  ParamDataTypeStr=Inherit: Same as input
  Integrator1 : Integrator
  Kp_c : Gain  Gain=Kp_c  SaturateOnIntegerOverflow=on  OutDataTypeStr=Inherit: Same as input  ParamDataTypeStr=Inherit: Same as input
  Normalize : Gain  Gain=1/v_max_c  SaturateOnIntegerOverflow=on  OutDataTypeStr=Inherit: Same as input  ParamDataTypeStr=Inherit: Same as input
  Normalize1 : Gain  Gain=1/v_max_c  SaturateOnIntegerOverflow=on  OutDataTypeStr=Inherit: Same as input  ParamDataTypeStr=Inherit: Same as input
  Sum1 : Sum  SaturateOnIntegerOverflow=on  InputSameDT=on  OutDataTypeStr=Inherit: Same as first input
  Sum5 : Sum  Inputs=-+  SaturateOnIntegerOverflow=on  InputSameDT=on  OutDataTypeStr=Inherit: Same as first input
  Sum7 : Sum  Inputs=+-  SaturateOnIntegerOverflow=on  InputSameDT=on  OutDataTypeStr=Inherit: Same as first input
  Sum8 : Sum  SaturateOnIntegerOverflow=on  InputSameDT=on  OutDataTypeStr=Inherit: Same as first input
  driver_cmd : Outport
  wires:
  Normalize1/1 -> Sum7/1
  v_veh/1 -> Normalize/1
  Normalize/1 -> Sum7/2
  v_des/1 -> Normalize1/1
  Sum5/1 -> 1/Tt_c/1
  "-1 to 1 "/1 -> Sum5/2, driver_cmd/1
  Integrator1/1 -> Sum1/2
  1/Ti_c/1 -> Sum8/1
  Sum8/1 -> Integrator1/1
  1/Tt_c/1 -> Sum8/2
  Kp_c/1 -> 1/Ti_c/1, Sum1/1
  Sum1/1 -> "-1 to 1 "/1, Sum5/1
  Sum7/1 -> Kp_c/1

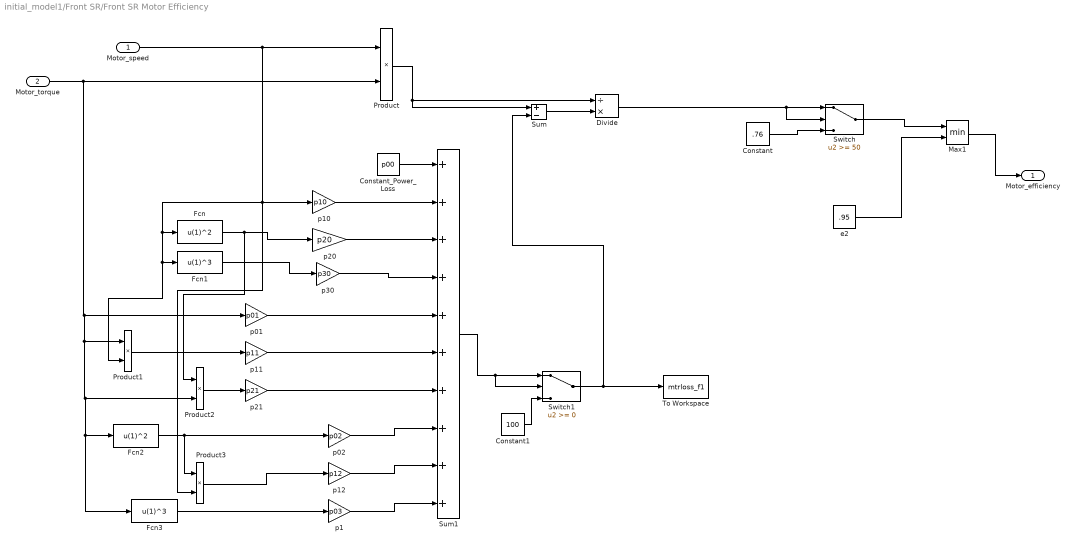
== system initial_model1/Front SR/Front SR Motor Efficiency ==
  Motor_speed : Inport
  Motor_torque : Inport  Port=2
  Constant : Constant  Value=.76
  Constant1 : Constant  Value=100
  Constant_Power_Loss : Constant  Value=p00
  Divide : Product  Inputs=/*
  Fcn : Fcn  Expr=u(1)^2
  Fcn1 : Fcn  Expr=u(1)^3
  Fcn2 : Fcn  Expr=u(1)^2
  Fcn3 : Fcn  Expr=u(1)^3
  Max1 : MinMax  Inputs=2
  Product{,1..3} (4 alike) : Product
  Sum : Sum  Inputs=+-
  Sum1 : Sum  Inputs=++++++++++
  Switch : Switch  Threshold=50
  Switch1 : Switch
  To Workspace : ToWorkspace  VariableName=mtrloss_f1  SampleTime=-1
      settings: MaxDataPoints=1  Save2DSignal=2-D array (concatenate along first dimension)
  e2 : Constant  Value=.95
  p01 : Gain  Gain=p01
  p02 : Gain  Gain=p02
  p1 : Gain  Gain=p03
  p10 : Gain  Gain=p10
  p11 : Gain  Gain=p11
  p12 : Gain  Gain=p12
  p20 : Gain  Gain=p20
  p21 : Gain  Gain=p21
  p30 : Gain  Gain=p30
  Motor_efficiency : Outport
  wires:
  Product3/1 -> p12/1
  Switch1/1 -> Sum/2, To Workspace/1
  Motor_torque/1 -> Product/2, p01/1, Product1/1, Product2/2, Fcn2/1, Fcn3/1
  Switch/1 -> Max1/1
  p10/1 -> Sum1/2
  p01/1 -> Sum1/5
  p1/1 -> Sum1/10
  Fcn3/1 -> p1/1
  p21/1 -> Sum1/7
  Constant_Power_Loss/1 -> Sum1/1
  Sum/1 -> Divide/2
  Product2/1 -> p21/1
  Motor_speed/1 -> Product/1, p10/1, Fcn/1, Fcn1/1, Product1/2, Product3/2
  Max1/1 -> Motor_efficiency/1
  Product1/1 -> p11/1
  Constant/1 -> Switch/3
  e2/1 -> Max1/2
  p20/1 -> Sum1/3
  p02/1 -> Sum1/8
  Product/1 -> Divide/1, Sum/1
  Fcn2/1 -> p02/1, Product3/1
  Fcn1/1 -> p30/1
  Sum1/1 -> Switch1/2, Switch1/1
  p30/1 -> Sum1/4
  Fcn/1 -> p20/1, Product2/1
  Constant1/1 -> Switch1/3
  p11/1 -> Sum1/6
  p12/1 -> Sum1/9
  Divide/1 -> Switch/1, Switch/2

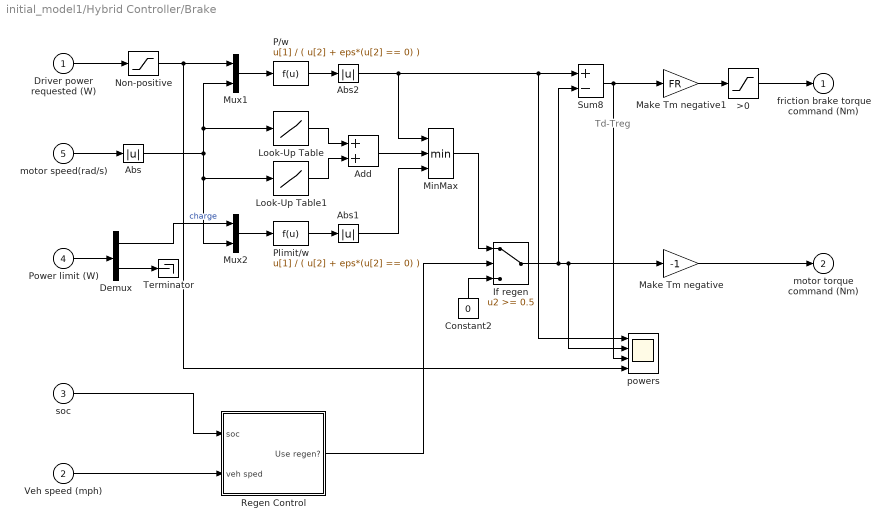
== system initial_model1/Hybrid Controller/Brake ==
  note: Td-Treg
  Driver power requested (W) : Inport
  Veh speed (mph) : Inport  Port=2
  soc : Inport  Port=3
  Power limit (W) : Inport  Port=4
  motor speed(rad/s) : Inport  Port=5
  >0 : Saturate  UpperLimit=10000  LowerLimit=0
  Abs : Abs  SaturateOnIntegerOverflow=on
  Abs1 : Abs  SaturateOnIntegerOverflow=on
  Abs2 : Abs  SaturateOnIntegerOverflow=on
  Add : Sum
  Constant2 : Constant  Value=0
  Demux : Demux  Outputs=2
  If regen : Switch  Threshold=0.5  SaturateOnIntegerOverflow=on  InputSameDT=on
  Look-Up Table : Lookup  InputValues=m_map_spd  Table=m_max_trq_SR  SaturateOnIntegerOverflow=on
  Look-Up Table1 : Lookup  InputValues=m_map_spd  Table=m_max_trq_IM  SaturateOnIntegerOverflow=on
  Make Tm negative : Gain  Gain=-1  SaturateOnIntegerOverflow=on  OutDataTypeStr=Inherit: Same as input  ParamDataTypeStr=Inherit: Same as input
  Make Tm negative1 : Gain  Gain=FR  SaturateOnIntegerOverflow=on  OutDataTypeStr=Inherit: Same as input  ParamDataTypeStr=Inherit: Same as input
  MinMax : MinMax  Inputs=3  SaturateOnIntegerOverflow=on  InputSameDT=on
  Mux1 : Mux  Inputs=2
  Mux2 : Mux  Inputs=2
  Non-positive : Saturate  UpperLimit=0  LowerLimit=-inf
  P/w : Fcn  Expr=u[1] / ( u[2] + eps*(u[2] == 0) )
  Plimit/w : Fcn  Expr=u[1] / ( u[2] + eps*(u[2] == 0) )
  Regen Control : Subsystem
      mask Display: disp('Regen\nControl')
  Sum8 : Sum  Inputs=+-  SaturateOnIntegerOverflow=on  InputSameDT=on  OutDataTypeStr=Inherit: Same as first input
  Terminator : Terminator
  powers : Scope  NumInputPorts=4
  friction brake torque command (Nm) : Outport
  motor torque command (Nm) : Outport  Port=2
  wires:
  Mux1/1 -> P/w/1
  Non-positive/1 -> Mux1/1, powers/4
  P/w/1 -> Abs2/1
  Constant2/1 -> If regen/3
  MinMax/1 -> If regen/1
  Demux/1 -> Mux2/1  "charge"
  Power limit (W)/1 -> Demux/1
  If regen/1 -> Make Tm negative/1, powers/2, Sum8/2
  Abs2/1 -> MinMax/1, Sum8/1, powers/1
  motor speed(rad/s)/1 -> Abs/1
  Abs/1 -> Look-Up Table/1, Mux1/2, Look-Up Table1/1, Mux2/2
  Make Tm negative1/1 -> >0/1
  Sum8/1 -> Make Tm negative1/1, powers/3
  Veh speed (mph)/1 -> Regen Control/2(veh sped)
  Plimit/w/1 -> Abs1/1
  Abs1/1 -> MinMax/3
  Driver power requested (W)/1 -> Non-positive/1
  soc/1 -> Regen Control/1(soc)
  >0/1 -> friction brake torque command (Nm)/1
  Make Tm negative/1 -> motor torque command (Nm)/1
  Mux2/1 -> Plimit/w/1
  Demux/2 -> Terminator/1
  Regen Control/1("Use regen? ") -> If regen/2
  Look-Up Table1/1 -> Add/2
  Look-Up Table/1 -> Add/1
  Add/1 -> MinMax/2

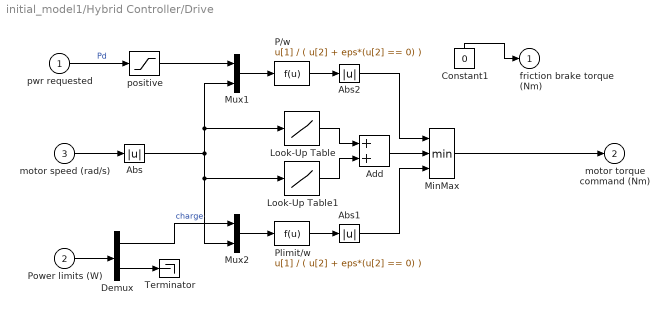
== system initial_model1/Hybrid Controller/Drive ==
  pwr requested : Inport
  Power limits (W) : Inport  Port=2
  motor speed (rad/s) : Inport  Port=3
  Abs : Abs  SaturateOnIntegerOverflow=on
  Abs1 : Abs  SaturateOnIntegerOverflow=on
  Abs2 : Abs  SaturateOnIntegerOverflow=on
  Add : Sum
  Constant1 : Constant  Value=0
  Demux : Demux  Outputs=2
  Look-Up Table : Lookup  InputValues=m_map_spd  Table=m_max_trq_SR  SaturateOnIntegerOverflow=on
  Look-Up Table1 : Lookup  InputValues=m_map_spd  Table=m_max_trq_IM  SaturateOnIntegerOverflow=on
  MinMax : MinMax  Inputs=3  SaturateOnIntegerOverflow=on  InputSameDT=on
  Mux1 : Mux  Inputs=2
  Mux2 : Mux  Inputs=2
  P/w : Fcn  Expr=u[1] / ( u[2] + eps*(u[2] == 0) )
  Plimit/w : Fcn  Expr=u[1] / ( u[2] + eps*(u[2] == 0) )
  Terminator : Terminator
  positive : Saturate  UpperLimit=inf  LowerLimit=0
  friction brake torque (Nm) : Outport
  motor torque command (Nm) : Outport  Port=2
  wires:
  Mux1/1 -> P/w/1
  positive/1 -> Mux1/1
  P/w/1 -> Abs2/1
  MinMax/1 -> motor torque command (Nm)/1
  Demux/1 -> Mux2/1  "charge"
  Power limits (W)/1 -> Demux/1
  Abs2/1 -> MinMax/1
  motor speed (rad/s)/1 -> Abs/1
  Plimit/w/1 -> Abs1/1
  Abs1/1 -> MinMax/3
  pwr requested/1 -> positive/1  "Pd"
  Mux2/1 -> Plimit/w/1
  Demux/2 -> Terminator/1
  Constant1/1 -> friction brake torque (Nm)/1
  Look-Up Table1/1 -> Add/2
  Look-Up Table/1 -> Add/1
  Abs/1 -> Look-Up Table/1, Mux1/2, Look-Up Table1/1, Mux2/2
  Add/1 -> MinMax/2

== system initial_model1/Hybrid Controller/pwr_demand ==
  note: max_brake_power
  note: >0:acc; <0:brake
  Accel cmd : Inport
  Decel cmd : Inport  Port=2
  Constant : Constant  Value=m_peak_pwr*1000
  Max braking torqu : Gain  Gain=200000  SaturateOnIntegerOverflow=on  OutDataTypeStr=Inherit: Same as input  ParamDataTypeStr=Inherit: Same as input
  Product : Product  SaturateOnIntegerOverflow=on  InputSameDT=on  OutDataTypeStr=Inherit: Same as first input
  Sum6 : Sum  Inputs=|+-  SaturateOnIntegerOverflow=on  InputSameDT=on  OutDataTypeStr=Inherit: Same as first input
  powers : Scope  NumInputPorts=3
  pwr dmd (W) : Outport
  wires:
  Decel cmd/1 -> Max braking torqu/1, powers/3
  Accel cmd/1 -> Product/2, powers/2
  Product/1 -> Sum6/1
  Max braking torqu/1 -> Sum6/2
  Constant/1 -> Product/1  "Max Driving Power"
  Sum6/1 -> pwr dmd (W)/1, powers/1

== system initial_model1/Rear IM/2 Speed Transmission Efficiency Decision ==
  Constant2 : Constant  Value=K_factor_in
  K_factor_out : Outport
  wires:
  Constant2/1 -> K_factor_out/1

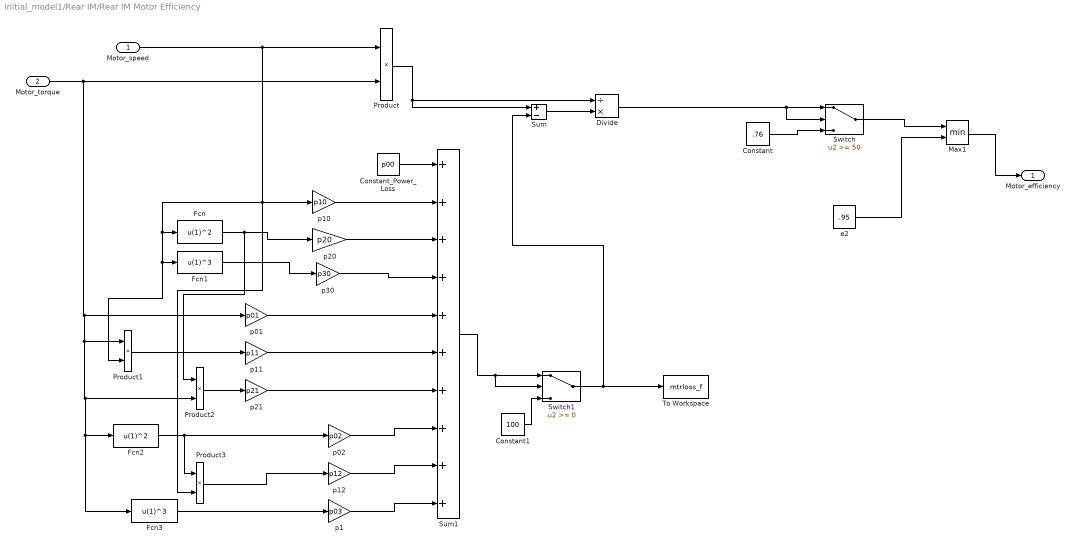
== system initial_model1/Rear IM/Rear IM Motor Efficiency ==
  Motor_speed : Inport
  Motor_torque : Inport  Port=2
  Constant : Constant  Value=.76
  Constant1 : Constant  Value=100
  Constant_Power_Loss : Constant  Value=p00
  Divide : Product  Inputs=/*
  Fcn : Fcn  Expr=u(1)^2
  Fcn1 : Fcn  Expr=u(1)^3
  Fcn2 : Fcn  Expr=u(1)^2
  Fcn3 : Fcn  Expr=u(1)^3
  Max1 : MinMax  Inputs=2
  Product{,1..3} (4 alike) : Product
  Sum : Sum  Inputs=+-
  Sum1 : Sum  Inputs=++++++++++
  Switch : Switch  Threshold=50
  Switch1 : Switch
  To Workspace : ToWorkspace  VariableName=mtrloss_f  SampleTime=-1
      settings: MaxDataPoints=1  Save2DSignal=2-D array (concatenate along first dimension)
  e2 : Constant  Value=.95
  p01 : Gain  Gain=p01
  p02 : Gain  Gain=p02
  p1 : Gain  Gain=p03
  p10 : Gain  Gain=p10
  p11 : Gain  Gain=p11
  p12 : Gain  Gain=p12
  p20 : Gain  Gain=p20
  p21 : Gain  Gain=p21
  p30 : Gain  Gain=p30
  Motor_efficiency : Outport
  wires:
  Product3/1 -> p12/1
  Switch1/1 -> Sum/2, To Workspace/1
  Motor_torque/1 -> Product/2, p01/1, Product1/1, Product2/2, Fcn2/1, Fcn3/1
  Switch/1 -> Max1/1
  p10/1 -> Sum1/2
  p01/1 -> Sum1/5
  p1/1 -> Sum1/10
  Fcn3/1 -> p1/1
  p21/1 -> Sum1/7
  Constant_Power_Loss/1 -> Sum1/1
  Sum/1 -> Divide/2
  Product2/1 -> p21/1
  Motor_speed/1 -> Product/1, p10/1, Fcn/1, Fcn1/1, Product1/2, Product3/2
  Max1/1 -> Motor_efficiency/1
  Product1/1 -> p11/1
  Constant/1 -> Switch/3
  e2/1 -> Max1/2
  p20/1 -> Sum1/3
  p02/1 -> Sum1/8
  Product/1 -> Divide/1, Sum/1
  Fcn2/1 -> p02/1, Product3/1
  Fcn1/1 -> p30/1
  Sum1/1 -> Switch1/2, Switch1/1
  p30/1 -> Sum1/4
  Fcn/1 -> p20/1, Product2/1
  Constant1/1 -> Switch1/3
  p11/1 -> Sum1/6
  p12/1 -> Sum1/9
  Divide/1 -> Switch/1, Switch/2

== system initial_model1/Vehicle/Dynamics ==
  note: Assumptions:
      | 1. No loss
      | 2. Small pinion gear inertia
      | 3. Longitudinal dynamics only
  wheel speed (rad/s) : Inport
  Tm: motor torque (N/m) : Inport  Port=2
  "Tfb: friction brake torque (N/m) " : Inport  Port=3
  Aero Drag : Fcn  Expr=0.5*A_frontal*rho_air* C_d*u^2*R_tire^3/FR^2
  Constant : Constant
  Constant1 : Constant  Value=0
  Gain : Gain  Gain=FR  SaturateOnIntegerOverflow=on  OutDataTypeStr=Inherit: Same as input  ParamDataTypeStr=Inherit: Same as input
  Integrator1 : Integrator  InitialCondition=0.1  LimitOutput=on  LowerSaturationLimit=0.1
  Rolling Resistance : Fcn  Expr=M_total*g_gravity*f_rolling*R_tire*u
  Sum : Sum  Inputs=+---  SaturateOnIntegerOverflow=on
  Switch : Switch  Threshold=0.001  SaturateOnIntegerOverflow=on
  To Workspace3 : ToWorkspace  VariableName=T_fb  SampleTime=-1
  Vehicle Propulsion : Fcn  Expr=u/(M_total*R_tire^2/FR)
  motor speed (rad/s) : Outport  InitialOutput=0
  wires:
  Vehicle Propulsion/1 -> Integrator1/1
  Integrator1/1 -> motor speed (rad/s)/1, Aero Drag/1
  Rolling Resistance/1 -> Sum/3  "Roll Resis"
  Aero Drag/1 -> Sum/4
  wheel speed (rad/s)/1 -> Switch/2
  Tm: motor torque (N/m)/1 -> Gain/1  "Tm"
  Constant1/1 -> Switch/3
  Constant/1 -> Switch/1
  Switch/1 -> Rolling Resistance/1
  Gain/1 -> Sum/1
  "Tfb: friction brake torque (N/m) "/1 -> Sum/2, To Workspace3/1  "Tf"
  Sum/1 -> Vehicle Propulsion/1

== system initial_model1/Battery/pack Voc, Rint/Rchg (ohms) ==
  x0 : Inport
  y0 : Inport  Port=2
  Mux : Mux  Inputs=2
  S-function : S-Function  FunctionName=sftable2  Parameters=xindex, yindex, table  SFunctionDeploymentMode=off  EnableBusSupport=off
  table out : Outport  InitialOutput=0
  wires:
  y0/1 -> Mux/2
  S-function/1 -> table out/1
  x0/1 -> Mux/1
  Mux/1 -> S-function/1

== system initial_model1/Battery/pack Voc, Rint/Rdis (ohms) ==
  x0 : Inport
  y0 : Inport  Port=2
  Mux : Mux  Inputs=2
  S-function : S-Function  FunctionName=sftable2  Parameters=xindex, yindex, table  SFunctionDeploymentMode=off  EnableBusSupport=off
  table out : Outport  InitialOutput=0
  wires:
  y0/1 -> Mux/2
  S-function/1 -> table out/1
  x0/1 -> Mux/1
  Mux/1 -> S-function/1

== system initial_model1/Battery/pack Voc, Rint/VOC (V) ==
  x0 : Inport
  y0 : Inport  Port=2
  Mux : Mux  Inputs=2
  S-function : S-Function  FunctionName=sftable2  Parameters=xindex, yindex, table  SFunctionDeploymentMode=off  EnableBusSupport=off
  table out : Outport  InitialOutput=0
  wires:
  y0/1 -> Mux/2
  S-function/1 -> table out/1
  x0/1 -> Mux/1
  Mux/1 -> S-function/1

== system initial_model1/Hybrid Controller/Brake/Regen Control ==
  soc : Inport
  veh sped : Inport  Port=2
  Logical Operator : Logic  Inputs=3
  regen swith on : Constant
  soc < soc_stopcharging : Relay  OnSwitchValue=regstop_soc  OffSwitchValue=regstop_soc  OnOutputValue=0  OffOutputValue=1
  veh spd>= 0.4 mph : Relay  OnSwitchValue=0.4  OffSwitchValue=0.4
  "Use regen? " : Outport
  wires:
  veh sped/1 -> veh spd>= 0.4 mph/1
  soc/1 -> soc < soc_stopcharging/1
  veh spd>= 0.4 mph/1 -> Logical Operator/1
  Logical Operator/1 -> "Use regen? "/1
  soc < soc_stopcharging/1 -> Logical Operator/2
  regen swith on/1 -> Logical Operator/3
